simulink model "lab"  (R2014b)
settings: Solver=ode45  StartTime=0.0  StopTime=250  RelTol=1e-3
settings Model: Creator=Student  LastModifiedBy=Student

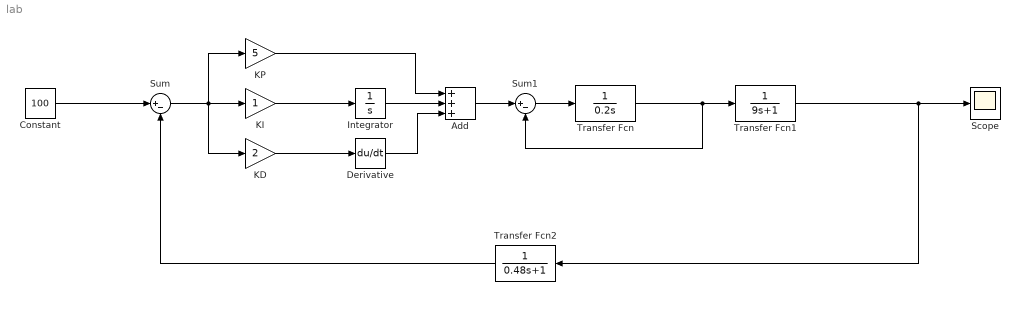
== system lab ==
  Add : Sum  Inputs=+++
  Constant : Constant  Value=100
  Derivative : Derivative
  Integrator : Integrator
  KD : Gain  Gain=2
  KI : Gain
  KP : Gain  Gain=5
  Scope : Scope
  Sum : Sum  Inputs=|+-
  Sum1 : Sum  Inputs=|+-
  Transfer Fcn : TransferFcn  Denominator=[0.2 0]
  Transfer Fcn1 : TransferFcn  Denominator=[9 +1]
  Transfer Fcn2 : TransferFcn  Denominator=[0.48 +1]
  wires:
  Constant/1 -> Sum/1
  Sum/1 -> KP/1, KI/1, KD/1
  KI/1 -> Integrator/1
  KD/1 -> Derivative/1
  Derivative/1 -> Add/3
  Integrator/1 -> Add/2
  KP/1 -> Add/1
  Add/1 -> Sum1/1
  Sum1/1 -> Transfer Fcn/1
  Transfer Fcn/1 -> Sum1/2, Transfer Fcn1/1
  Transfer Fcn2/1 -> Sum/2
  Transfer Fcn1/1 -> Transfer Fcn2/1, Scope/1
